simulink model "fuel_injector"  (R2014b)
settings: Solver=ode3  StartTime=0.0  StopTime=10.0  FixedStep=10  RelTol=1e-3
values from neighbouring files (symbols this model uses):
  m_dot_fc_test = m_dot_fc(k)    [testfile.m]
  N_test = N(k)    [testfile.m]
  t_inj_test = t_inj(k)    [testfile.m]
undefined symbols (not defined in the file or in its folder): c_fi, n_cyl, n_r, t_0
settings Model: Creator=danfa688  LastModifiedBy=danfa688

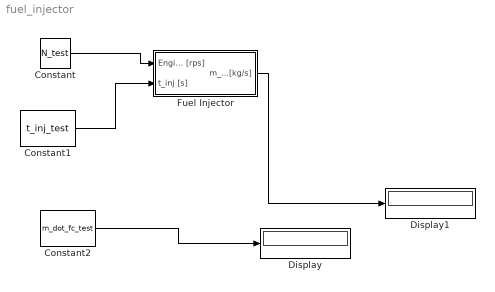
== system fuel_injector ==
  Constant : Constant  Value=N_test
  Constant1 : Constant  Value=t_inj_test
  Constant2 : Constant  Value=m_dot_fc_test
  Display : Display
  Display1 : Display
  Fuel Injector : Subsystem
  wires:
  Fuel Injector/1(m_dot_fc [kg/s]) -> Display1/1
  Constant/1 -> Fuel Injector/1(Engine Speed [rps])
  Constant1/1 -> Fuel Injector/2(t_inj [s])
  Constant2/1 -> Display/1

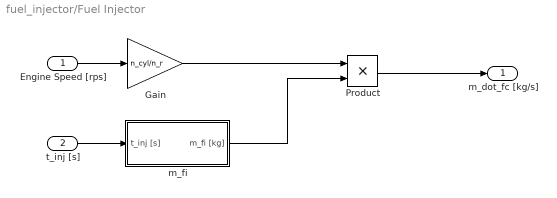
== system fuel_injector/Fuel Injector ==
  Engine Speed [rps] : Inport
  t_inj [s] : Inport  Port=2
  Gain : Gain  Gain=n_cyl/n_r
  Product : Product
  m_fi : Subsystem
  m_dot_fc [kg/s] : Outport
  wires:
  t_inj [s]/1 -> m_fi/1(t_inj [s])
  m_fi/1(m_fi [kg]) -> Product/2
  Engine Speed [rps]/1 -> Gain/1
  Gain/1 -> Product/1
  Product/1 -> m_dot_fc [kg/s]/1

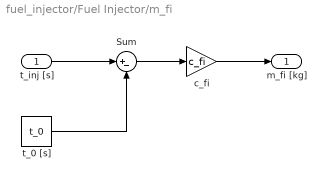
== system fuel_injector/Fuel Injector/m_fi ==
  t_inj [s] : Inport
  Sum : Sum  Inputs=|+-
  c_fi : Gain  Gain=c_fi
  t_0 [s] : Constant  Value=t_0
  m_fi [kg] : Outport
  wires:
  t_0 [s]/1 -> Sum/2
  t_inj [s]/1 -> Sum/1
  Sum/1 -> c_fi/1
  c_fi/1 -> m_fi [kg]/1
